simulink model "ad9361_sim"  (R2014a)
settings: Solver=ode45  StartTime=0.0  StopTime=Inf  RelTol=1e-3
libraries: dspsrcs4 x2, simulink x2
settings Model: Creator=ACozma  LastModifiedBy=ACozma
settings DebuggingCC: UnderspecifiedInitializationDetection=Classic

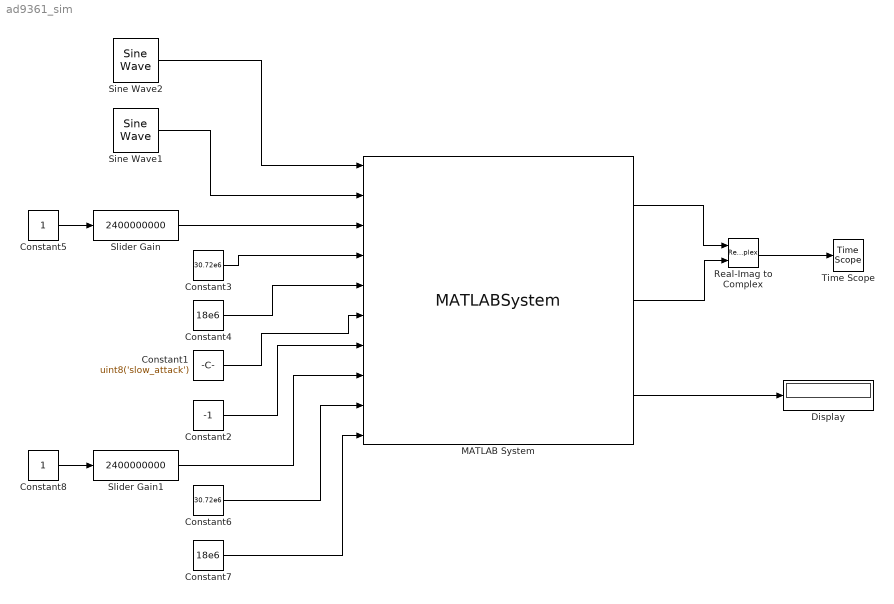
== system ad9361_sim ==
  Constant1 : Constant  Value=uint8('slow_attack')
  Constant2 : Constant  Value=-1
  Constant3 : Constant  Value=30.72e6
  Constant4 : Constant  Value=18e6
  Constant5 : Constant
  Constant6 : Constant  Value=30.72e6
  Constant7 : Constant  Value=18e6
  Constant8 : Constant
  Display : Display
  MATLAB System : MATLABSystem  DialogController=sysobjdialog.BlockDynDialog  System=iio_sys_obj  SimulateUsing=Interpreted execution  ip_address=10.50.1.147  dev_name=ad9361  in_ch_no=2  in_ch_size=32768  out_ch_no=2  out_ch_size=8192
      mask Type: iio_sys_obj
      mask Display:
      | disp('ad9361');
      | port_label('input',1,'DATA_IN1');
      | port_label('input',2,'DATA_IN2');
      | port_label('input',3,'RX_LO_FREQ');
      | port_label('input',4,'RX_SAMPLING_FREQ');
      | port_label('input',5,'RX_RF_BANDWIDTH');
      | port_label('input',6,'RX1_GAIN_MODE');
      | port_label('input',7,'RX1_GAIN');
      | port_label('input',8,'TX_LO_FREQ');
      | port_label('input',9,'TX_SAMPLING_FREQ');
      | port_label('input',10,'TX_RF_BANDWIDTH');
      | port_label('output',1,'DATA_OUT1');
      | port_label('output',2,'DATA_OUT2');
      | port_label('output',3,'RX1_RSSI');
  Real-Imag to Complex : RealImagToComplex
  Sine Wave1 : dspsrcs4/Sine Wave  Amplitude=32768  Frequency=100  Phase=pi/2  SampleMode=Discrete  OutComplex=Real  CompMethod=Trigonometric fcn  TableSize=Speed  SampleTime=1/10000  SamplesPerFrame=32768  ResetState=Catch up to simulation time  dataType=double  wordLen=16  udDataType=sfix(16)  fracBitsMode=Best precision  numFracBits=15  OutDataTypeStr=double  LastOutDataTypeStr=double
  Sine Wave2 : dspsrcs4/Sine Wave  Amplitude=32768  Frequency=100  Phase=0  SampleMode=Discrete  OutComplex=Real  CompMethod=Trigonometric fcn  TableSize=Speed  SampleTime=1/10000  SamplesPerFrame=32768  ResetState=Catch up to simulation time  dataType=double  wordLen=16  udDataType=sfix(16)  fracBitsMode=Best precision  numFracBits=15  OutDataTypeStr=double  LastOutDataTypeStr=double
  Slider Gain : simulink/Math Operations/Slider Gain  low=200000  gain=2400000000  high=6000000000
  Slider Gain1 : simulink/Math Operations/Slider Gain  low=200000  gain=2400000000  high=6000000000
  Time Scope : TimeScope  DefaultConfigurationName=spbscopes.TimeScopeBlockCfg
  wires:
  Slider Gain/1 -> MATLAB System/3
  Constant3/1 -> MATLAB System/4
  Constant4/1 -> MATLAB System/5
  Constant1/1 -> MATLAB System/6
  Constant2/1 -> MATLAB System/7
  Slider Gain1/1 -> MATLAB System/8
  Constant5/1 -> Slider Gain/1
  Constant8/1 -> Slider Gain1/1
  Constant6/1 -> MATLAB System/9
  Constant7/1 -> MATLAB System/10
  MATLAB System/3 -> Display/1
  MATLAB System/1 -> Real-Imag to Complex/1
  MATLAB System/2 -> Real-Imag to Complex/2
  Sine Wave2/1 -> MATLAB System/1
  Sine Wave1/1 -> MATLAB System/2
  Real-Imag to Complex/1 -> Time Scope/1
